simulink model "Complex_Real_Imag"  (R2020a)
settings: Solver=VariableStepAuto  StartTime=0.0  StopTime=10.0  RelTol=1e-3
settings Model: Creator=royde  LastModifiedBy=royde

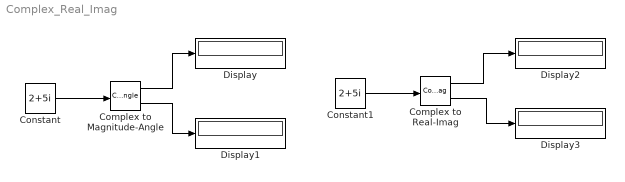
== system Complex_Real_Imag ==
  Complex to Magnitude-Angle : ComplexToMagnitudeAngle
  Complex to Real-Imag : ComplexToRealImag
  Constant : Constant  Value=2+5i
  Constant1 : Constant  Value=2+5i
  Display{,1..3} (4 alike) : Display
  wires:
  Constant/1 -> Complex to Magnitude-Angle/1
  Constant1/1 -> Complex to Real-Imag/1
  Complex to Magnitude-Angle/1 -> Display/1
  Complex to Magnitude-Angle/2 -> Display1/1
  Complex to Real-Imag/2 -> Display3/1
  Complex to Real-Imag/1 -> Display2/1
